simulink model "SSN_39busRT_Ctrl_4WT_19B"  (R2021a)
settings: Solver=ode3  StartTime=0.0  StopTime=10  FixedStep=Ts  MaxStep=1/60  RelTol=1e-2  AbsTol=1e-1
PreLoadFcn:
  | Ts=2.50e-6; ssn_ieee39_params; load('Pwf.mat');
InitFcn:
  | Ts=2.50e-6; ssn_ieee39_params; load('Pwf.mat');
values from neighbouring files (symbols this model uses):
  f = 50    [ssn_ieee39_params_ctrl.m]
  fNom = f    (= 60)    [ssn_ieee39_params_ctrl.m]
  ILR = 5.02    [ssn_ieee39_params_ctrl.m]
  IQMIN = 0.1    [ssn_ieee39_params_ctrl.m]
  ISCLIM = 1    [ssn_ieee39_params_ctrl.m]
  ITFpu = 1.10    (= 1.1)    [ssn_ieee39_params_ctrl.m]
  K = 1    [ssn_ieee39_params_ctrl.m]
  K1 = 1    [ssn_ieee39_params_ctrl.m]
  K2 = 2    [ssn_ieee39_params_ctrl.m]
  KCL = 1.04    [ssn_ieee39_params_ctrl.m]
  KFB = 0    [ssn_ieee39_params_ctrl.m]
  KFF = 1    [ssn_ieee39_params_ctrl.m]
  KFIX = 1    [ssn_ieee39_params_ctrl.m]
  KG = 1    [ssn_ieee39_params_ctrl.m]
  KIA = 59.91    [ssn_ieee39_params_ctrl.m]
  KIOEX = 0.0303    [ssn_ieee39_params_ctrl.m]
  KIUEX = 0.0303    [ssn_ieee39_params_ctrl.m]
  KIUOEX = 1    [ssn_ieee39_params_ctrl.m]
  KIUUEX = 1    [ssn_ieee39_params_ctrl.m]
  KLR = 22.47    [ssn_ieee39_params_ctrl.m]
  KM = 1    [ssn_ieee39_params_ctrl.m]
  KOEL = 0.24    [ssn_ieee39_params_ctrl.m]
  Kp = 1    [ssn_ieee39_params_ctrl.m]
  KPA = 30    [ssn_ieee39_params_ctrl.m]
  KPOEL = 1    [ssn_ieee39_params_ctrl.m]
  KPOEX = 0    [ssn_ieee39_params_ctrl.m]
  KPUEX = 0    [ssn_ieee39_params_ctrl.m]
  KSCALE = 0.319    [ssn_ieee39_params_ctrl.m]
  KUF = 0    [ssn_ieee39_params_ctrl.m]
  KUI = 0.001    [ssn_ieee39_params_ctrl.m]
  KUL = 0.24    [ssn_ieee39_params_ctrl.m]
  s = 10    [ssn_ieee39_params_ctrl.m]
  TA = 0.01    [ssn_ieee39_params_ctrl.m]
  Tadj = 0    [ssn_ieee39_params_ctrl.m]
  taps = [1 1 1.07 1.07 1.009 1.025 1 1.025 1.025 1.025]*1    [ssn_ieee39_params_ctrl.m]
  TF = 0.02    [ssn_ieee39_params_ctrl.m]
  TG = 0.024    [ssn_ieee39_params_ctrl.m]
  TINV = 0    [ssn_ieee39_params_ctrl.m]
  TIT = 0.1    [ssn_ieee39_params_ctrl.m]
  TL_10_11_len = 14    [ssn_ieee39_params_ctrl.m]
  TL_10_13_len = 14    [ssn_ieee39_params_ctrl.m]
  TL_13_14_len = 32    [ssn_ieee39_params_ctrl.m]
  TL_14_15_len = 70    [ssn_ieee39_params_ctrl.m]
  TL_15_16_len = 31.5    [ssn_ieee39_params_ctrl.m]
  TL_16_17_len = 26    [ssn_ieee39_params_ctrl.m]
  TL_16_19_len = 61    [ssn_ieee39_params_ctrl.m]
  TL_16_21_len = 46    [ssn_ieee39_params_ctrl.m]
  TL_16_24_len = 15    [ssn_ieee39_params_ctrl.m]
  TL_17_18_len = 26    [ssn_ieee39_params_ctrl.m]
  TL_17_27_len = 59    [ssn_ieee39_params_ctrl.m]
  TL_1_2_len = 134    [ssn_ieee39_params_ctrl.m]
  TL_1_39_len = 105    [ssn_ieee39_params_ctrl.m]
  TL_21_22_len = 47    [ssn_ieee39_params_ctrl.m]
  TL_22_23_len = 33    [ssn_ieee39_params_ctrl.m]
  TL_24_23_len = 88    [ssn_ieee39_params_ctrl.m]
  TL_25_26_len = 101    [ssn_ieee39_params_ctrl.m]
  TL_26_27_len = 46.5    [ssn_ieee39_params_ctrl.m]
  TL_26_28_len = 151    [ssn_ieee39_params_ctrl.m]
  TL_26_29_len = 200    [ssn_ieee39_params_ctrl.m]
  TL_28_29_len = 48    [ssn_ieee39_params_ctrl.m]
  TL_2_25_len = 28    [ssn_ieee39_params_ctrl.m]
  TL_2_2_len = 49    [ssn_ieee39_params_ctrl.m]
  TL_3_18_len = 42    [ssn_ieee39_params_ctrl.m]
  TL_3_4_len = 53    [ssn_ieee39_params_ctrl.m]
  TL_4_14_len = 33    [ssn_ieee39_params_ctrl.m]
  TL_4_5_len = 32.5    [ssn_ieee39_params_ctrl.m]
  TL_5_6_len = 14    [ssn_ieee39_params_ctrl.m]
  TL_5_8_len = 32    [ssn_ieee39_params_ctrl.m]
  TL_6_11_len = 26.5    [ssn_ieee39_params_ctrl.m]
  TL_6_7_len = 25.5    [ssn_ieee39_params_ctrl.m]
  TL_7_8_len = 15    [ssn_ieee39_params_ctrl.m]
  TL_8_9_len = 93    [ssn_ieee39_params_ctrl.m]
  TL_9_39_len = 136    [ssn_ieee39_params_ctrl.m]
  TOEL = 5.00    (= 5)    [ssn_ieee39_params_ctrl.m]
  TQREF = 0    [ssn_ieee39_params_ctrl.m]
  TQSCL = 0.012    [ssn_ieee39_params_ctrl.m]
  Ts_PMU = 1/1000    (= 0.001)    [ssn_ieee39_params_ctrl.m]
  TU1 = 0    [ssn_ieee39_params_ctrl.m]
  TU2 = 0    [ssn_ieee39_params_ctrl.m]
  TU3 = 0    [ssn_ieee39_params_ctrl.m]
  TU4 = 0    [ssn_ieee39_params_ctrl.m]
  TUL = 0    [ssn_ieee39_params_ctrl.m]
  TUP = 0.050    (= 0.05)    [ssn_ieee39_params_ctrl.m]
  TUQ = .005    (= 0.005)    [ssn_ieee39_params_ctrl.m]
  TUV = 0.2    [ssn_ieee39_params_ctrl.m]
  VAAMAX = VAMAX    (= 7.05)    [ssn_ieee39_params_ctrl.m]
  VAMAX = 7.05    [ssn_ieee39_params_ctrl.m]
  VAMIN = -6.11    [ssn_ieee39_params_ctrl.m]
  VBMAX = 999    [ssn_ieee39_params_ctrl.m]
  VF = 0    [ssn_ieee39_params_ctrl.m]
  VFB = 0    [ssn_ieee39_params_ctrl.m]
  VMMAX = 7.05    [ssn_ieee39_params_ctrl.m]
  VMMIN = -6.11    [ssn_ieee39_params_ctrl.m]
  VOELmax1 = 0.2353    [ssn_ieee39_params_ctrl.m]
  VOELmax2 = 0.0    (= 0)    [ssn_ieee39_params_ctrl.m]
  VOELmin1 = -0.24    [ssn_ieee39_params_ctrl.m]
  VOELmin2 = -1.0    (= -1)    [ssn_ieee39_params_ctrl.m]
  VRMAX = 7.05    [ssn_ieee39_params_ctrl.m]
  VRMIN = -6.11    [ssn_ieee39_params_ctrl.m]
  VSCLmax = 0.20    (= 0.2)    [ssn_ieee39_params_ctrl.m]
  VSCLmin = -0.10    (= -0.1)    [ssn_ieee39_params_ctrl.m]
  VUELmax1 = 1    [ssn_ieee39_params_ctrl.m]
  VUELmax2 = 1    [ssn_ieee39_params_ctrl.m]
  VUELmin1 = -1    [ssn_ieee39_params_ctrl.m]
  VUELmin2 = -1    [ssn_ieee39_params_ctrl.m]
  VUImax = 1    [ssn_ieee39_params_ctrl.m]
  VUImin = -1    [ssn_ieee39_params_ctrl.m]
undefined symbols (not defined in the file or in its folder): another_event_name, D1, Delta, DiscIntNeverNeededParam, find_system, MOV_segment9, my_event_name, powergui, Pw1, Pw2, Pw3, Pw4, vNomHV
libraries: powerlib_extras x162, spsThreePhaseVIMeasurementLib x55, spsCurrentMeasurementLib x52, simulink_extras x44, slpidlib x40, op_dpl_lib x36, spsST2AModel x20, spsThreePhaseParallelRLCLoadLib x20, spsThreePhaseTransformerTwoWindingsLib x17, spsControlledVoltageSourceLib x16, spsVoltageMeasurementLib x12, spsSynchronousMachinepuStandardLib x10
(part 16 of 19)

== system SSN_39busRT_Ctrl_4WT_19B/SM_master/4 WT/SS_windfarm3to4/Wind Farm (DFIG Type)/Wind Turbine Doubly-Fed Induction Generator (Average Model)1/Average_VSC/Converter_model ==
  note: P = Vab*Ia -Vbc*Ic = Vdc*Idc
      | Idc = (Vab*Ia -Vbc*Ic)/Vdc
  Ia_Ic : Inport
  Vdc : Inport  Port=2
  Uref : Inport  Port=3
  Add : Sum  Inputs=+-
  Add1 : Sum  Inputs=+-
  Constant : Constant  Value=1e-6
  Delay1 : UnitDelay  SampleTime=Ts  HasFrameUpgradeWarning=on
  Delay2 : UnitDelay  InitialCondition=1e-6  SampleTime=Ts  HasFrameUpgradeWarning=on
  Demux : Demux  Outputs=3
  Demux1 : Demux  Outputs=2
  Gain : Gain  Gain=0.5
  Mult : Product  Inputs=**
  Mux1 : Mux  Inputs=2
  Predictor : Subsystem
  Product3 : Product  RndMeth=Zero
  Product4 : Product  RndMeth=Zero
  Product5 : Product  Inputs=*/  RndMeth=Zero
  Subtract2 : Sum  Inputs=+-
  Subtract3 : Sum
  Idc : Outport
  Vab_Vbc : Outport  Port=2
  wires:
  Delay1/1 -> Gain/1, Predictor/1(In)
  Gain/1 -> Mult/2
  Mult/1 -> Demux/1
  Demux/3 -> Add1/2
  Demux/2 -> Add/2, Add1/1
  Demux/1 -> Add/1
  Predictor/1(Out) -> Subtract3/1
  Add/1 -> Mux1/1, Product3/1  "Vab"
  Add1/1 -> Mux1/2, Product4/1  "Vbc"
  Demux1/2 -> Product4/2  "ic"
  Product3/1 -> Subtract2/1
  Product4/1 -> Subtract2/2
  Subtract3/1 -> Product5/2
  Constant/1 -> Subtract3/2
  Product5/1 -> Delay2/1
  Subtract2/1 -> Product5/1  "Pac"
  Demux1/1 -> Product3/2  "ia"
  Delay2/1 -> Idc/1  "idc"
  Ia_Ic/1 -> Demux1/1
  Vdc/1 -> Delay1/1
  Uref/1 -> Mult/1
  Mux1/1 -> Vab_Vbc/1

== system SSN_39busRT_Ctrl_4WT_19B/SM_master/4 WT/SS_windfarm3to4/Wind Farm (DFIG Type)/Wind Turbine Doubly-Fed Induction Generator (Average Model)1/Average_VSC1/Converter_model ==
  note: P = Vab*Ia -Vbc*Ic = Vdc*Idc
      | Idc = (Vab*Ia -Vbc*Ic)/Vdc
  Ia_Ic : Inport
  Vdc : Inport  Port=2
  Uref : Inport  Port=3
  Add : Sum  Inputs=+-
  Add1 : Sum  Inputs=+-
  Constant : Constant  Value=1e-6
  Delay1 : UnitDelay  SampleTime=Ts  HasFrameUpgradeWarning=on
  Delay2 : UnitDelay  InitialCondition=1e-6  SampleTime=Ts  HasFrameUpgradeWarning=on
  Demux : Demux  Outputs=3
  Demux1 : Demux  Outputs=2
  Gain : Gain  Gain=0.5
  Mult : Product  Inputs=**
  Mux1 : Mux  Inputs=2
  Predictor : Subsystem
  Product3 : Product  RndMeth=Zero
  Product4 : Product  RndMeth=Zero
  Product5 : Product  Inputs=*/  RndMeth=Zero
  Subtract2 : Sum  Inputs=+-
  Subtract3 : Sum
  Idc : Outport
  Vab_Vbc : Outport  Port=2
  wires:
  Delay1/1 -> Gain/1, Predictor/1(In)
  Gain/1 -> Mult/2
  Mult/1 -> Demux/1
  Demux/3 -> Add1/2
  Demux/2 -> Add/2, Add1/1
  Demux/1 -> Add/1
  Predictor/1(Out) -> Subtract3/1
  Add/1 -> Mux1/1, Product3/1  "Vab"
  Add1/1 -> Mux1/2, Product4/1  "Vbc"
  Demux1/2 -> Product4/2  "ic"
  Product3/1 -> Subtract2/1
  Product4/1 -> Subtract2/2
  Subtract3/1 -> Product5/2
  Constant/1 -> Subtract3/2
  Product5/1 -> Delay2/1
  Subtract2/1 -> Product5/1  "Pac"
  Demux1/1 -> Product3/2  "ia"
  Delay2/1 -> Idc/1  "idc"
  Ia_Ic/1 -> Demux1/1
  Vdc/1 -> Delay1/1
  Uref/1 -> Mult/1
  Mux1/1 -> Vab_Vbc/1

== system SSN_39busRT_Ctrl_4WT_19B/SM_master/4 WT/SS_windfarm3to4/Wind Farm (DFIG Type)/Wind Turbine Doubly-Fed Induction Generator (Average Model)1/Control System_average/Control ==
  Vabc_B1 : Inport
  Iabc_grid_conv : Inport  Port=2
  Vdc : Inport  Port=3
  Iabc_stator : Inport  Port=4
  Iabc_rotor : Inport  Port=5
  Q_ref : Inport  Port=6
  Iq_grid_conv_ref : Inport  Port=7
  Q_B1 : Inport  Port=8
  wr : Inport  Port=9
  angle_rotor : Inport  Port=10
  0-pitch_max : Saturate  UpperLimit=pitch_max  LowerLimit=0
  Constant2 : Constant  Value=speed_D
  Discrete 3-phase PLL : powerlib_extras/Discrete  Control Blocks/Discrete 3-phase PLL  Fmin=Fnom-10  Par_Init=[-45 Fnom]  ParK=[60 1400]  Ts=Ts  AGC=off
      settings: SourceProductBaseCode=PS
  Grid-side converter Control system : Subsystem
  Mux : Mux  Inputs=2
  "Rate Limiter   " : RateLimiter  RisingSlewLimit=pitch_rate  FallingSlewLimit=-pitch_rate
  Rotor-side converter Control system : Subsystem
  Sum : Sum  Inputs=|+-  SaturateOnIntegerOverflow=on
  Terminator : Terminator
  pitch_gain : Gain  Gain=pitch_gain  SaturateOnIntegerOverflow=on  OutDataTypeStr=Inherit: Same as input  ParamDataTypeStr=Inherit: Same as input
  Uctrl_grid_conv : Outport
  Uctrl_rotor_conv : Outport  Port=2
  Theta_Freq : Outport  Port=3
  Pitch_angle : Outport  Port=4
  wires:
  Vdc/1 -> Grid-side converter Control system/4(Vdc), Rotor-side converter Control system/2(Vdc)
  Vabc_B1/1 -> Grid-side converter Control system/1(Vabc_B1), Discrete 3-phase PLL/1
  Iq_grid_conv_ref/1 -> Grid-side converter Control system/5(Iq_ref)
  Iabc_grid_conv/1 -> Grid-side converter Control system/2(Iabc_grid_conv), Rotor-side converter Control system/6(Iabc_grid_conv)
  Iabc_stator/1 -> Rotor-side converter Control system/4(Iabc_stator)
  Iabc_rotor/1 -> Rotor-side converter Control system/5(Iabc_rotor)
  Q_ref/1 -> Rotor-side converter Control system/7(Q_ref)
  Discrete 3-phase PLL/2 -> Grid-side converter Control system/3(Theta), Mux/1, Rotor-side converter Control system/3(Theta)
  Mux/1 -> Theta_Freq/1
  Discrete 3-phase PLL/3 -> Terminator/1
  Discrete 3-phase PLL/1 -> Grid-side converter Control system/6(Freq), Mux/2, Rotor-side converter Control system/10(Freq)
  "Rate Limiter   "/1 -> Pitch_angle/1
  pitch_gain/1 -> 0-pitch_max/1
  Sum/1 -> pitch_gain/1
  Constant2/1 -> Sum/2
  0-pitch_max/1 -> "Rate Limiter   "/1
  wr/1 -> Sum/1, Rotor-side converter Control system/1(wr)
  Q_B1/1 -> Rotor-side converter Control system/8(Q_B1)
  angle_rotor/1 -> Rotor-side converter Control system/9(angle_rotor)
  Grid-side converter Control system/2(Vdqs) -> [Vdqs]
  [Vdqs] -> Rotor-side converter Control system/11(Vdqs)
  Grid-side converter Control system/1(Uctrl_grid_conv) -> Uctrl_grid_conv/1
  Rotor-side converter Control system/1(Uctrl_rotor_conv) -> Uctrl_rotor_conv/1

== system SSN_39busRT_Ctrl_4WT_19B/SM_master/4 WT/SS_windfarm3to4/Wind Farm (DFIG Type)/Wind Turbine Doubly-Fed Induction Generator (Average Model)1/Control System_average/Filter 1000 Hz ==
  Vabc_B1 : Inport
  Iabc_grid_conv : Inport  Port=2
  Vdc : Inport  Port=3
  Iabc_stator : Inport  Port=4
  Iabc_rotor : Inport  Port=5
  Q_ref : Inport  Port=6
  Iq_grid_conv_ref : Inport  Port=7
  Q_B1 : Inport  Port=8
  wr : Inport  Port=9
  angle_rotor : Inport  Port=10
  Demux{,1..3} (4 alike) : Demux  Outputs=3
      settings: DisplayOption=none
  Discrete 2nd-Order Filter{1..14,16..18,20} (18 alike) : powerlib_extras/Discrete  Control Blocks/Discrete  2nd-Order Filter  FilterType=Lowpass  Fo=Freq  Zeta=Zeta  Ts=Ts  Initialize=off  Vac_Init=[0.8 -25 60]  Vdc_Init=-0.4  PlotResponse=off  param1=[1 500 1]
      settings: SourceProductBaseCode=PS
  Mux{,1..3} (4 alike) : Mux  Inputs=3
  "Vabc_B1 " : Outport
  "Iabc_grid_conv " : Outport  Port=2
  "Vdc " : Outport  Port=3
  "Iabc_stator " : Outport  Port=4
  "Iabc_rotor " : Outport  Port=5
  "Q_ref " : Outport  Port=6
  "Iq_grid_conv_ref " : Outport  Port=7
  "Q_B1 " : Outport  Port=8
  "wr " : Outport  Port=9
  "angle_rotor " : Outport  Port=10
  wires:
  Demux/1 -> Discrete 2nd-Order Filter1/1
  Demux/2 -> Discrete 2nd-Order Filter2/1
  Demux/3 -> Discrete 2nd-Order Filter3/1
  Discrete 2nd-Order Filter1/1 -> Mux/1
  Discrete 2nd-Order Filter2/1 -> Mux/2
  Discrete 2nd-Order Filter3/1 -> Mux/3
  Vabc_B1/1 -> Demux/1
  Mux/1 -> "Vabc_B1 "/1
  Demux1/1 -> Discrete 2nd-Order Filter4/1
  Demux1/2 -> Discrete 2nd-Order Filter5/1
  Demux1/3 -> Discrete 2nd-Order Filter6/1
  Discrete 2nd-Order Filter4/1 -> Mux1/1
  Discrete 2nd-Order Filter5/1 -> Mux1/2
  Discrete 2nd-Order Filter6/1 -> Mux1/3
  Iabc_grid_conv/1 -> Demux1/1
  Mux1/1 -> "Iabc_grid_conv "/1
  Vdc/1 -> Discrete 2nd-Order Filter7/1
  Discrete 2nd-Order Filter7/1 -> "Vdc "/1
  Demux2/1 -> Discrete 2nd-Order Filter8/1
  Demux2/2 -> Discrete 2nd-Order Filter9/1
  Demux2/3 -> Discrete 2nd-Order Filter10/1
  Discrete 2nd-Order Filter8/1 -> Mux2/1
  Discrete 2nd-Order Filter9/1 -> Mux2/2
  Discrete 2nd-Order Filter10/1 -> Mux2/3
  Iabc_stator/1 -> Demux2/1
  Mux2/1 -> "Iabc_stator "/1
  Q_ref/1 -> Discrete 2nd-Order Filter11/1
  Q_B1/1 -> Discrete 2nd-Order Filter12/1
  Discrete 2nd-Order Filter12/1 -> "Q_B1 "/1
  wr/1 -> Discrete 2nd-Order Filter13/1
  Discrete 2nd-Order Filter13/1 -> "wr "/1
  angle_rotor/1 -> Discrete 2nd-Order Filter14/1
  Discrete 2nd-Order Filter14/1 -> "angle_rotor "/1
  Discrete 2nd-Order Filter11/1 -> "Q_ref "/1
  Demux3/1 -> Discrete 2nd-Order Filter17/1
  Demux3/2 -> Discrete 2nd-Order Filter18/1
  Demux3/3 -> Discrete 2nd-Order Filter16/1
  Discrete 2nd-Order Filter17/1 -> Mux3/1
  Discrete 2nd-Order Filter18/1 -> Mux3/2
  Discrete 2nd-Order Filter16/1 -> Mux3/3
  Iabc_rotor/1 -> Demux3/1
  Mux3/1 -> "Iabc_rotor "/1
  Iq_grid_conv_ref/1 -> Discrete 2nd-Order Filter20/1
  Discrete 2nd-Order Filter20/1 -> "Iq_grid_conv_ref "/1

== system SSN_39busRT_Ctrl_4WT_19B/SM_master/4 WT/SS_windfarm3to4/Wind Farm (DFIG Type)2/Wind Turbine Doubly-Fed Induction Generator (Average Model)1/Average_VSC/Converter_model ==
  note: P = Vab*Ia -Vbc*Ic = Vdc*Idc
      | Idc = (Vab*Ia -Vbc*Ic)/Vdc
  Ia_Ic : Inport
  Vdc : Inport  Port=2
  Uref : Inport  Port=3
  Add : Sum  Inputs=+-
  Add1 : Sum  Inputs=+-
  Constant : Constant  Value=1e-6
  Delay1 : UnitDelay  SampleTime=Ts  HasFrameUpgradeWarning=on
  Delay2 : UnitDelay  InitialCondition=1e-6  SampleTime=Ts  HasFrameUpgradeWarning=on
  Demux : Demux  Outputs=3
  Demux1 : Demux  Outputs=2
  Gain : Gain  Gain=0.5
  Mult : Product  Inputs=**
  Mux1 : Mux  Inputs=2
  Predictor : Subsystem
  Product3 : Product  RndMeth=Zero
  Product4 : Product  RndMeth=Zero
  Product5 : Product  Inputs=*/  RndMeth=Zero
  Subtract2 : Sum  Inputs=+-
  Subtract3 : Sum
  Idc : Outport
  Vab_Vbc : Outport  Port=2
  wires:
  Mux1/1 -> Vab_Vbc/1
  Uref/1 -> Mult/1
  Vdc/1 -> Delay1/1
  Ia_Ic/1 -> Demux1/1
  Delay2/1 -> Idc/1  "idc"
  Demux1/1 -> Product3/2  "ia"
  Subtract2/1 -> Product5/1  "Pac"
  Product5/1 -> Delay2/1
  Constant/1 -> Subtract3/2
  Subtract3/1 -> Product5/2
  Product4/1 -> Subtract2/2
  Product3/1 -> Subtract2/1
  Demux1/2 -> Product4/2  "ic"
  Add1/1 -> Product4/1, Mux1/2  "Vbc"
  Add/1 -> Product3/1, Mux1/1  "Vab"
  Predictor/1(Out) -> Subtract3/1
  Demux/1 -> Add/1
  Demux/2 -> Add1/1, Add/2
  Demux/3 -> Add1/2
  Mult/1 -> Demux/1
  Gain/1 -> Mult/2
  Delay1/1 -> Predictor/1(In), Gain/1

== system SSN_39busRT_Ctrl_4WT_19B/SM_master/4 WT/SS_windfarm3to4/Wind Farm (DFIG Type)2/Wind Turbine Doubly-Fed Induction Generator (Average Model)1/Average_VSC1/Converter_model ==
  note: P = Vab*Ia -Vbc*Ic = Vdc*Idc
      | Idc = (Vab*Ia -Vbc*Ic)/Vdc
  Ia_Ic : Inport
  Vdc : Inport  Port=2
  Uref : Inport  Port=3
  Add : Sum  Inputs=+-
  Add1 : Sum  Inputs=+-
  Constant : Constant  Value=1e-6
  Delay1 : UnitDelay  SampleTime=Ts  HasFrameUpgradeWarning=on
  Delay2 : UnitDelay  InitialCondition=1e-6  SampleTime=Ts  HasFrameUpgradeWarning=on
  Demux : Demux  Outputs=3
  Demux1 : Demux  Outputs=2
  Gain : Gain  Gain=0.5
  Mult : Product  Inputs=**
  Mux1 : Mux  Inputs=2
  Predictor : Subsystem
  Product3 : Product  RndMeth=Zero
  Product4 : Product  RndMeth=Zero
  Product5 : Product  Inputs=*/  RndMeth=Zero
  Subtract2 : Sum  Inputs=+-
  Subtract3 : Sum
  Idc : Outport
  Vab_Vbc : Outport  Port=2
  wires:
  Mux1/1 -> Vab_Vbc/1
  Uref/1 -> Mult/1
  Vdc/1 -> Delay1/1
  Ia_Ic/1 -> Demux1/1
  Delay2/1 -> Idc/1  "idc"
  Demux1/1 -> Product3/2  "ia"
  Subtract2/1 -> Product5/1  "Pac"
  Product5/1 -> Delay2/1
  Constant/1 -> Subtract3/2
  Subtract3/1 -> Product5/2
  Product4/1 -> Subtract2/2
  Product3/1 -> Subtract2/1
  Demux1/2 -> Product4/2  "ic"
  Add1/1 -> Product4/1, Mux1/2  "Vbc"
  Add/1 -> Product3/1, Mux1/1  "Vab"
  Predictor/1(Out) -> Subtract3/1
  Demux/1 -> Add/1
  Demux/2 -> Add1/1, Add/2
  Demux/3 -> Add1/2
  Mult/1 -> Demux/1
  Gain/1 -> Mult/2
  Delay1/1 -> Predictor/1(In), Gain/1

== system SSN_39busRT_Ctrl_4WT_19B/SM_master/4 WT/SS_windfarm3to4/Wind Farm (DFIG Type)2/Wind Turbine Doubly-Fed Induction Generator (Average Model)1/Control System_average/Control ==
  Vabc_B1 : Inport
  Iabc_grid_conv : Inport  Port=2
  Vdc : Inport  Port=3
  Iabc_stator : Inport  Port=4
  Iabc_rotor : Inport  Port=5
  Q_ref : Inport  Port=6
  Iq_grid_conv_ref : Inport  Port=7
  Q_B1 : Inport  Port=8
  wr : Inport  Port=9
  angle_rotor : Inport  Port=10
  0-pitch_max : Saturate  UpperLimit=pitch_max  LowerLimit=0
  Constant2 : Constant  Value=speed_D
  Discrete 3-phase PLL : powerlib_extras/Discrete  Control Blocks/Discrete 3-phase PLL  Fmin=Fnom-10  Par_Init=[-45 Fnom]  ParK=[60 1400]  Ts=Ts  AGC=off
      settings: SourceProductBaseCode=PS
  Grid-side converter Control system : Subsystem
  Mux : Mux  Inputs=2
  "Rate Limiter   " : RateLimiter  RisingSlewLimit=pitch_rate  FallingSlewLimit=-pitch_rate
  Rotor-side converter Control system : Subsystem
  Sum : Sum  Inputs=|+-  SaturateOnIntegerOverflow=on
  Terminator : Terminator
  pitch_gain : Gain  Gain=pitch_gain  SaturateOnIntegerOverflow=on  OutDataTypeStr=Inherit: Same as input  ParamDataTypeStr=Inherit: Same as input
  Uctrl_grid_conv : Outport
  Uctrl_rotor_conv : Outport  Port=2
  Theta_Freq : Outport  Port=3
  Pitch_angle : Outport  Port=4
  wires:
  Rotor-side converter Control system/1(Uctrl_rotor_conv) -> Uctrl_rotor_conv/1
  Grid-side converter Control system/1(Uctrl_grid_conv) -> Uctrl_grid_conv/1
  [Vdqs] -> Rotor-side converter Control system/11(Vdqs)
  Grid-side converter Control system/2(Vdqs) -> [Vdqs]
  angle_rotor/1 -> Rotor-side converter Control system/9(angle_rotor)
  Q_B1/1 -> Rotor-side converter Control system/8(Q_B1)
  wr/1 -> Rotor-side converter Control system/1(wr), Sum/1
  0-pitch_max/1 -> "Rate Limiter   "/1
  Constant2/1 -> Sum/2
  Sum/1 -> pitch_gain/1
  pitch_gain/1 -> 0-pitch_max/1
  "Rate Limiter   "/1 -> Pitch_angle/1
  Discrete 3-phase PLL/1 -> Rotor-side converter Control system/10(Freq), Mux/2, Grid-side converter Control system/6(Freq)
  Discrete 3-phase PLL/3 -> Terminator/1
  Mux/1 -> Theta_Freq/1
  Discrete 3-phase PLL/2 -> Rotor-side converter Control system/3(Theta), Mux/1, Grid-side converter Control system/3(Theta)
  Q_ref/1 -> Rotor-side converter Control system/7(Q_ref)
  Iabc_rotor/1 -> Rotor-side converter Control system/5(Iabc_rotor)
  Iabc_stator/1 -> Rotor-side converter Control system/4(Iabc_stator)
  Iabc_grid_conv/1 -> Rotor-side converter Control system/6(Iabc_grid_conv), Grid-side converter Control system/2(Iabc_grid_conv)
  Iq_grid_conv_ref/1 -> Grid-side converter Control system/5(Iq_ref)
  Vabc_B1/1 -> Discrete 3-phase PLL/1, Grid-side converter Control system/1(Vabc_B1)
  Vdc/1 -> Rotor-side converter Control system/2(Vdc), Grid-side converter Control system/4(Vdc)

== system SSN_39busRT_Ctrl_4WT_19B/SM_master/4 WT/SS_windfarm3to4/Wind Farm (DFIG Type)2/Wind Turbine Doubly-Fed Induction Generator (Average Model)1/Control System_average/Filter 1000 Hz ==
  Vabc_B1 : Inport
  Iabc_grid_conv : Inport  Port=2
  Vdc : Inport  Port=3
  Iabc_stator : Inport  Port=4
  Iabc_rotor : Inport  Port=5
  Q_ref : Inport  Port=6
  Iq_grid_conv_ref : Inport  Port=7
  Q_B1 : Inport  Port=8
  wr : Inport  Port=9
  angle_rotor : Inport  Port=10
  Demux{,1..3} (4 alike) : Demux  Outputs=3
      settings: DisplayOption=none
  Discrete 2nd-Order Filter{1..14,16..18,20} (18 alike) : powerlib_extras/Discrete  Control Blocks/Discrete  2nd-Order Filter  FilterType=Lowpass  Fo=Freq  Zeta=Zeta  Ts=Ts  Initialize=off  Vac_Init=[0.8 -25 60]  Vdc_Init=-0.4  PlotResponse=off  param1=[1 500 1]
      settings: SourceProductBaseCode=PS
  Mux{,1..3} (4 alike) : Mux  Inputs=3
  "Vabc_B1 " : Outport
  "Iabc_grid_conv " : Outport  Port=2
  "Vdc " : Outport  Port=3
  "Iabc_stator " : Outport  Port=4
  "Iabc_rotor " : Outport  Port=5
  "Q_ref " : Outport  Port=6
  "Iq_grid_conv_ref " : Outport  Port=7
  "Q_B1 " : Outport  Port=8
  "wr " : Outport  Port=9
  "angle_rotor " : Outport  Port=10
  wires:
  Discrete 2nd-Order Filter20/1 -> "Iq_grid_conv_ref "/1
  Iq_grid_conv_ref/1 -> Discrete 2nd-Order Filter20/1
  Mux3/1 -> "Iabc_rotor "/1
  Iabc_rotor/1 -> Demux3/1
  Discrete 2nd-Order Filter16/1 -> Mux3/3
  Discrete 2nd-Order Filter18/1 -> Mux3/2
  Discrete 2nd-Order Filter17/1 -> Mux3/1
  Demux3/3 -> Discrete 2nd-Order Filter16/1
  Demux3/2 -> Discrete 2nd-Order Filter18/1
  Demux3/1 -> Discrete 2nd-Order Filter17/1
  Discrete 2nd-Order Filter11/1 -> "Q_ref "/1
  Discrete 2nd-Order Filter14/1 -> "angle_rotor "/1
  angle_rotor/1 -> Discrete 2nd-Order Filter14/1
  Discrete 2nd-Order Filter13/1 -> "wr "/1
  wr/1 -> Discrete 2nd-Order Filter13/1
  Discrete 2nd-Order Filter12/1 -> "Q_B1 "/1
  Q_B1/1 -> Discrete 2nd-Order Filter12/1
  Q_ref/1 -> Discrete 2nd-Order Filter11/1
  Mux2/1 -> "Iabc_stator "/1
  Iabc_stator/1 -> Demux2/1
  Discrete 2nd-Order Filter10/1 -> Mux2/3
  Discrete 2nd-Order Filter9/1 -> Mux2/2
  Discrete 2nd-Order Filter8/1 -> Mux2/1
  Demux2/3 -> Discrete 2nd-Order Filter10/1
  Demux2/2 -> Discrete 2nd-Order Filter9/1
  Demux2/1 -> Discrete 2nd-Order Filter8/1
  Discrete 2nd-Order Filter7/1 -> "Vdc "/1
  Vdc/1 -> Discrete 2nd-Order Filter7/1
  Mux1/1 -> "Iabc_grid_conv "/1
  Iabc_grid_conv/1 -> Demux1/1
  Discrete 2nd-Order Filter6/1 -> Mux1/3
  Discrete 2nd-Order Filter5/1 -> Mux1/2
  Discrete 2nd-Order Filter4/1 -> Mux1/1
  Demux1/3 -> Discrete 2nd-Order Filter6/1
  Demux1/2 -> Discrete 2nd-Order Filter5/1
  Demux1/1 -> Discrete 2nd-Order Filter4/1
  Mux/1 -> "Vabc_B1 "/1
  Vabc_B1/1 -> Demux/1
  Discrete 2nd-Order Filter3/1 -> Mux/3
  Discrete 2nd-Order Filter2/1 -> Mux/2
  Discrete 2nd-Order Filter1/1 -> Mux/1
  Demux/3 -> Discrete 2nd-Order Filter3/1
  Demux/2 -> Discrete 2nd-Order Filter2/1
  Demux/1 -> Discrete 2nd-Order Filter1/1

== system SSN_39busRT_Ctrl_4WT_19B/SM_master/4 WT/SS_windfarm1to2/Wind Farm (DFIG Type)/Wind Turbine Doubly-Fed Induction Generator (Average Model)1/Average_VSC/Converter_model/Predictor ==
  In : Inport
  Add2 : Sum  Inputs=+-
  Gain1 : Gain  Gain=2
  Unit Delay : UnitDelay  SampleTime=Ts  HasFrameUpgradeWarning=on
  Out : Outport
  wires:
  In/1 -> Unit Delay/1, Gain1/1
  Gain1/1 -> Add2/1
  Unit Delay/1 -> Add2/2
  Add2/1 -> Out/1

== system SSN_39busRT_Ctrl_4WT_19B/SM_master/4 WT/SS_windfarm1to2/Wind Farm (DFIG Type)/Wind Turbine Doubly-Fed Induction Generator (Average Model)1/Average_VSC1/Converter_model/Predictor ==
  In : Inport
  Add2 : Sum  Inputs=+-
  Gain1 : Gain  Gain=2
  Unit Delay : UnitDelay  SampleTime=Ts  HasFrameUpgradeWarning=on
  Out : Outport
  wires:
  In/1 -> Unit Delay/1, Gain1/1
  Gain1/1 -> Add2/1
  Unit Delay/1 -> Add2/2
  Add2/1 -> Out/1

== system SSN_39busRT_Ctrl_4WT_19B/SM_master/4 WT/SS_windfarm1to2/Wind Farm (DFIG Type)/Wind Turbine Doubly-Fed Induction Generator (Average Model)1/Control System_average/Control/Grid-side converter Control system ==
  note: Grid-side converter control system
  Vabc_B1 : Inport
  Iabc_grid_conv : Inport  Port=2
  Theta : Inport  Port=3
  Vdc : Inport  Port=4
  Iq_ref : Inport  Port=5
  Freq : Inport  Port=6
  Current regulator : Subsystem
  DC bus voltage Regulator : Subsystem
  Idq references : Subsystem
  Mux : Mux  Inputs=2
  Rate Limiter : RateLimiter  RisingSlewLimit=current_slew_rate  FallingSlewLimit=-current_slew_rate
  Subsystem1 : Subsystem
  Transformation abc --> dq : Subsystem
  Vdc_ref (V) : Constant  Value=Vdc_nom
  Uctrl_grid_conv : Outport
  Vdqs : Outport  Port=2
  wires:
  Transformation abc --> dq/1(Vdq) -> Current regulator/1(Vdqs), Vdqs/1
  Theta/1 -> Transformation abc --> dq/1(Theta), Subsystem1/1(Theta)
  Vdc/1 -> Subsystem1/3(Vdc), DC bus voltage Regulator/2(Vdc)
  DC bus voltage Regulator/1(Id_ref) -> Mux/1
  Transformation abc --> dq/2(Idq) -> Current regulator/2(Idq)
  Mux/1 -> Idq references/1(Id*Iq*)
  Rate Limiter/1 -> Mux/2
  Iq_ref/1 -> Rate Limiter/1
  Vabc_B1/1 -> Transformation abc --> dq/2(Vabc)
  Iabc_grid_conv/1 -> Transformation abc --> dq/3(Iabc)
  Subsystem1/1(Uctrl_grid_conv) -> Uctrl_grid_conv/1
  Vdc_ref (V)/1 -> DC bus voltage Regulator/1(Vdc_ref)
  Current regulator/1(Vdq*) -> Subsystem1/2(Vdq*)
  Idq references/1(Idq_ref) -> Current regulator/4(Idq_ref)
  Freq/1 -> Current regulator/3(Freq)

== system SSN_39busRT_Ctrl_4WT_19B/SM_master/4 WT/SS_windfarm1to2/Wind Farm (DFIG Type)/Wind Turbine Doubly-Fed Induction Generator (Average Model)1/Control System_average/Control/Rotor-side converter Control system ==
  note: Rotor-side converter control system
  wr : Inport
  Vdc : Inport  Port=2
  Theta : Inport  Port=3
  Iabc_stator : Inport  Port=4
  Iabc_rotor : Inport  Port=5
  Iabc_grid_conv : Inport  Port=6
  Q_ref : Inport  Port=7
  Q_B1 : Inport  Port=8
  angle_rotor : Inport  Port=9
  Freq : Inport  Port=10
  Vdqs : Inport  Port=11
  Current Regulator : Subsystem
  Mux3 : Mux  Inputs=2
  Priority Iqr : Subsystem
  Q Regulator : Subsystem
  Torque control : Subsystem
  "Transformation abc --> dq " : Subsystem
  dq --> abc : Subsystem
  Uctrl_rotor_conv : Outport
  wires:
  Current Regulator/1(Vdq*) -> dq --> abc/1(Vdq*)
  Vdc/1 -> dq --> abc/2(Vdc)
  Theta/1 -> "Transformation abc --> dq "/1(Theta)
  dq --> abc/1(Uctrl_rotor_conv) -> Uctrl_rotor_conv/1
  Iabc_rotor/1 -> "Transformation abc --> dq "/2(Iabc_r)
  Iabc_stator/1 -> "Transformation abc --> dq "/3(Iabc_s)
  Iabc_grid_conv/1 -> "Transformation abc --> dq "/4(Iabc_grid_conv)
  "Transformation abc --> dq "/1(Idq_r) -> Current Regulator/2(Idq_r), Torque control/2(Idqr)
  "Transformation abc --> dq "/2(Idq_s) -> Torque control/3(Idqs), Current Regulator/3(Idq_s)
  angle_rotor/1 -> "Transformation abc --> dq "/5(angle_rotor)
  Mux3/1 -> Priority Iqr/1(Idqr*)
  "Transformation abc --> dq "/4(r_angle_transformation) -> dq --> abc/3(Angle)
  Freq/1 -> Torque control/5(Freq), Current Regulator/5(Freq)
  wr/1 -> Torque control/1(wr), Current Regulator/4(wr)
  "Transformation abc --> dq "/3(Idq_gc) -> Torque control/4(Idq_grid_conv)
  Vdqs/1 -> Torque control/6(Vdqs)
  Q_ref/1 -> Q Regulator/1(Q_ref)
  Q_B1/1 -> Q Regulator/2(Q_B1)
  Torque control/1(Idr*) -> Mux3/1
  Q Regulator/1(Iqr*) -> Mux3/2
  Priority Iqr/1(Idqr_ref) -> Current Regulator/1(Idqr_ref)

== system SSN_39busRT_Ctrl_4WT_19B/SM_master/4 WT/SS_windfarm1to2/Wind Farm (DFIG Type)1/Wind Turbine Doubly-Fed Induction Generator (Average Model)1/Average_VSC/Converter_model/Predictor ==
  In : Inport
  Add2 : Sum  Inputs=+-
  Gain1 : Gain  Gain=2
  Unit Delay : UnitDelay  SampleTime=Ts  HasFrameUpgradeWarning=on
  Out : Outport
  wires:
  Add2/1 -> Out/1
  Unit Delay/1 -> Add2/2
  Gain1/1 -> Add2/1
  In/1 -> Gain1/1, Unit Delay/1

== system SSN_39busRT_Ctrl_4WT_19B/SM_master/4 WT/SS_windfarm1to2/Wind Farm (DFIG Type)1/Wind Turbine Doubly-Fed Induction Generator (Average Model)1/Average_VSC1/Converter_model/Predictor ==
  In : Inport
  Add2 : Sum  Inputs=+-
  Gain1 : Gain  Gain=2
  Unit Delay : UnitDelay  SampleTime=Ts  HasFrameUpgradeWarning=on
  Out : Outport
  wires:
  Add2/1 -> Out/1
  Unit Delay/1 -> Add2/2
  Gain1/1 -> Add2/1
  In/1 -> Gain1/1, Unit Delay/1

== system SSN_39busRT_Ctrl_4WT_19B/SM_master/4 WT/SS_windfarm1to2/Wind Farm (DFIG Type)1/Wind Turbine Doubly-Fed Induction Generator (Average Model)1/Control System_average/Control/Grid-side converter Control system ==
  note: Grid-side converter control system
  Vabc_B1 : Inport
  Iabc_grid_conv : Inport  Port=2
  Theta : Inport  Port=3
  Vdc : Inport  Port=4
  Iq_ref : Inport  Port=5
  Freq : Inport  Port=6
  Current regulator : Subsystem
  DC bus voltage Regulator : Subsystem
  Idq references : Subsystem
  Mux : Mux  Inputs=2
  Rate Limiter : RateLimiter  RisingSlewLimit=current_slew_rate  FallingSlewLimit=-current_slew_rate
  Subsystem1 : Subsystem
  Transformation abc --> dq : Subsystem
  Vdc_ref (V) : Constant  Value=Vdc_nom
  Uctrl_grid_conv : Outport
  Vdqs : Outport  Port=2
  wires:
  Freq/1 -> Current regulator/3(Freq)
  Idq references/1(Idq_ref) -> Current regulator/4(Idq_ref)
  Current regulator/1(Vdq*) -> Subsystem1/2(Vdq*)
  Vdc_ref (V)/1 -> DC bus voltage Regulator/1(Vdc_ref)
  Subsystem1/1(Uctrl_grid_conv) -> Uctrl_grid_conv/1
  Iabc_grid_conv/1 -> Transformation abc --> dq/3(Iabc)
  Vabc_B1/1 -> Transformation abc --> dq/2(Vabc)
  Iq_ref/1 -> Rate Limiter/1
  Rate Limiter/1 -> Mux/2
  Mux/1 -> Idq references/1(Id*Iq*)
  Transformation abc --> dq/2(Idq) -> Current regulator/2(Idq)
  DC bus voltage Regulator/1(Id_ref) -> Mux/1
  Vdc/1 -> DC bus voltage Regulator/2(Vdc), Subsystem1/3(Vdc)
  Theta/1 -> Subsystem1/1(Theta), Transformation abc --> dq/1(Theta)
  Transformation abc --> dq/1(Vdq) -> Vdqs/1, Current regulator/1(Vdqs)

== system SSN_39busRT_Ctrl_4WT_19B/SM_master/4 WT/SS_windfarm1to2/Wind Farm (DFIG Type)1/Wind Turbine Doubly-Fed Induction Generator (Average Model)1/Control System_average/Control/Rotor-side converter Control system ==
  note: Rotor-side converter control system
  wr : Inport
  Vdc : Inport  Port=2
  Theta : Inport  Port=3
  Iabc_stator : Inport  Port=4
  Iabc_rotor : Inport  Port=5
  Iabc_grid_conv : Inport  Port=6
  Q_ref : Inport  Port=7
  Q_B1 : Inport  Port=8
  angle_rotor : Inport  Port=9
  Freq : Inport  Port=10
  Vdqs : Inport  Port=11
  Current Regulator : Subsystem
  Mux3 : Mux  Inputs=2
  Priority Iqr : Subsystem
  Q Regulator : Subsystem
  Torque control : Subsystem
  "Transformation abc --> dq " : Subsystem
  dq --> abc : Subsystem
  Uctrl_rotor_conv : Outport
  wires:
  Priority Iqr/1(Idqr_ref) -> Current Regulator/1(Idqr_ref)
  Q Regulator/1(Iqr*) -> Mux3/2
  Torque control/1(Idr*) -> Mux3/1
  Q_B1/1 -> Q Regulator/2(Q_B1)
  Q_ref/1 -> Q Regulator/1(Q_ref)
  Vdqs/1 -> Torque control/6(Vdqs)
  "Transformation abc --> dq "/3(Idq_gc) -> Torque control/4(Idq_grid_conv)
  wr/1 -> Current Regulator/4(wr), Torque control/1(wr)
  Freq/1 -> Current Regulator/5(Freq), Torque control/5(Freq)
  "Transformation abc --> dq "/4(r_angle_transformation) -> dq --> abc/3(Angle)
  Mux3/1 -> Priority Iqr/1(Idqr*)
  angle_rotor/1 -> "Transformation abc --> dq "/5(angle_rotor)
  "Transformation abc --> dq "/2(Idq_s) -> Current Regulator/3(Idq_s), Torque control/3(Idqs)
  "Transformation abc --> dq "/1(Idq_r) -> Torque control/2(Idqr), Current Regulator/2(Idq_r)
  Iabc_grid_conv/1 -> "Transformation abc --> dq "/4(Iabc_grid_conv)
  Iabc_stator/1 -> "Transformation abc --> dq "/3(Iabc_s)
  Iabc_rotor/1 -> "Transformation abc --> dq "/2(Iabc_r)
  dq --> abc/1(Uctrl_rotor_conv) -> Uctrl_rotor_conv/1
  Theta/1 -> "Transformation abc --> dq "/1(Theta)
  Vdc/1 -> dq --> abc/2(Vdc)
  Current Regulator/1(Vdq*) -> dq --> abc/1(Vdq*)

== system SSN_39busRT_Ctrl_4WT_19B/SM_master/4 WT/SS_windfarm3to4/Wind Farm (DFIG Type)/Wind Turbine Doubly-Fed Induction Generator (Average Model)1/Average_VSC/Converter_model/Predictor ==
  In : Inport
  Add2 : Sum  Inputs=+-
  Gain1 : Gain  Gain=2
  Unit Delay : UnitDelay  SampleTime=Ts  HasFrameUpgradeWarning=on
  Out : Outport
  wires:
  In/1 -> Unit Delay/1, Gain1/1
  Gain1/1 -> Add2/1
  Unit Delay/1 -> Add2/2
  Add2/1 -> Out/1

== system SSN_39busRT_Ctrl_4WT_19B/SM_master/4 WT/SS_windfarm3to4/Wind Farm (DFIG Type)/Wind Turbine Doubly-Fed Induction Generator (Average Model)1/Average_VSC1/Converter_model/Predictor ==
  In : Inport
  Add2 : Sum  Inputs=+-
  Gain1 : Gain  Gain=2
  Unit Delay : UnitDelay  SampleTime=Ts  HasFrameUpgradeWarning=on
  Out : Outport
  wires:
  In/1 -> Unit Delay/1, Gain1/1
  Gain1/1 -> Add2/1
  Unit Delay/1 -> Add2/2
  Add2/1 -> Out/1

== system SSN_39busRT_Ctrl_4WT_19B/SM_master/4 WT/SS_windfarm3to4/Wind Farm (DFIG Type)/Wind Turbine Doubly-Fed Induction Generator (Average Model)1/Control System_average/Control/Grid-side converter Control system ==
  note: Grid-side converter control system
  Vabc_B1 : Inport
  Iabc_grid_conv : Inport  Port=2
  Theta : Inport  Port=3
  Vdc : Inport  Port=4
  Iq_ref : Inport  Port=5
  Freq : Inport  Port=6
  Current regulator : Subsystem
  DC bus voltage Regulator : Subsystem
  Idq references : Subsystem
  Mux : Mux  Inputs=2
  Rate Limiter : RateLimiter  RisingSlewLimit=current_slew_rate  FallingSlewLimit=-current_slew_rate
  Subsystem1 : Subsystem
  Transformation abc --> dq : Subsystem
  Vdc_ref (V) : Constant  Value=Vdc_nom
  Uctrl_grid_conv : Outport
  Vdqs : Outport  Port=2
  wires:
  Transformation abc --> dq/1(Vdq) -> Current regulator/1(Vdqs), Vdqs/1
  Theta/1 -> Transformation abc --> dq/1(Theta), Subsystem1/1(Theta)
  Vdc/1 -> Subsystem1/3(Vdc), DC bus voltage Regulator/2(Vdc)
  DC bus voltage Regulator/1(Id_ref) -> Mux/1
  Transformation abc --> dq/2(Idq) -> Current regulator/2(Idq)
  Mux/1 -> Idq references/1(Id*Iq*)
  Rate Limiter/1 -> Mux/2
  Iq_ref/1 -> Rate Limiter/1
  Vabc_B1/1 -> Transformation abc --> dq/2(Vabc)
  Iabc_grid_conv/1 -> Transformation abc --> dq/3(Iabc)
  Subsystem1/1(Uctrl_grid_conv) -> Uctrl_grid_conv/1
  Vdc_ref (V)/1 -> DC bus voltage Regulator/1(Vdc_ref)
  Current regulator/1(Vdq*) -> Subsystem1/2(Vdq*)
  Idq references/1(Idq_ref) -> Current regulator/4(Idq_ref)
  Freq/1 -> Current regulator/3(Freq)

== system SSN_39busRT_Ctrl_4WT_19B/SM_master/4 WT/SS_windfarm3to4/Wind Farm (DFIG Type)/Wind Turbine Doubly-Fed Induction Generator (Average Model)1/Control System_average/Control/Rotor-side converter Control system ==
  note: Rotor-side converter control system
  wr : Inport
  Vdc : Inport  Port=2
  Theta : Inport  Port=3
  Iabc_stator : Inport  Port=4
  Iabc_rotor : Inport  Port=5
  Iabc_grid_conv : Inport  Port=6
  Q_ref : Inport  Port=7
  Q_B1 : Inport  Port=8
  angle_rotor : Inport  Port=9
  Freq : Inport  Port=10
  Vdqs : Inport  Port=11
  Current Regulator : Subsystem
  Mux3 : Mux  Inputs=2
  Priority Iqr : Subsystem
  Q Regulator : Subsystem
  Torque control : Subsystem
  "Transformation abc --> dq " : Subsystem
  dq --> abc : Subsystem
  Uctrl_rotor_conv : Outport
  wires:
  Current Regulator/1(Vdq*) -> dq --> abc/1(Vdq*)
  Vdc/1 -> dq --> abc/2(Vdc)
  Theta/1 -> "Transformation abc --> dq "/1(Theta)
  dq --> abc/1(Uctrl_rotor_conv) -> Uctrl_rotor_conv/1
  Iabc_rotor/1 -> "Transformation abc --> dq "/2(Iabc_r)
  Iabc_stator/1 -> "Transformation abc --> dq "/3(Iabc_s)
  Iabc_grid_conv/1 -> "Transformation abc --> dq "/4(Iabc_grid_conv)
  "Transformation abc --> dq "/1(Idq_r) -> Current Regulator/2(Idq_r), Torque control/2(Idqr)
  "Transformation abc --> dq "/2(Idq_s) -> Torque control/3(Idqs), Current Regulator/3(Idq_s)
  angle_rotor/1 -> "Transformation abc --> dq "/5(angle_rotor)
  Mux3/1 -> Priority Iqr/1(Idqr*)
  "Transformation abc --> dq "/4(r_angle_transformation) -> dq --> abc/3(Angle)
  Freq/1 -> Torque control/5(Freq), Current Regulator/5(Freq)
  wr/1 -> Torque control/1(wr), Current Regulator/4(wr)
  "Transformation abc --> dq "/3(Idq_gc) -> Torque control/4(Idq_grid_conv)
  Vdqs/1 -> Torque control/6(Vdqs)
  Q_ref/1 -> Q Regulator/1(Q_ref)
  Q_B1/1 -> Q Regulator/2(Q_B1)
  Torque control/1(Idr*) -> Mux3/1
  Q Regulator/1(Iqr*) -> Mux3/2
  Priority Iqr/1(Idqr_ref) -> Current Regulator/1(Idqr_ref)

== system SSN_39busRT_Ctrl_4WT_19B/SM_master/4 WT/SS_windfarm3to4/Wind Farm (DFIG Type)2/Wind Turbine Doubly-Fed Induction Generator (Average Model)1/Average_VSC/Converter_model/Predictor ==
  In : Inport
  Add2 : Sum  Inputs=+-
  Gain1 : Gain  Gain=2
  Unit Delay : UnitDelay  SampleTime=Ts  HasFrameUpgradeWarning=on
  Out : Outport
  wires:
  Add2/1 -> Out/1
  Unit Delay/1 -> Add2/2
  Gain1/1 -> Add2/1
  In/1 -> Gain1/1, Unit Delay/1

== system SSN_39busRT_Ctrl_4WT_19B/SM_master/4 WT/SS_windfarm3to4/Wind Farm (DFIG Type)2/Wind Turbine Doubly-Fed Induction Generator (Average Model)1/Average_VSC1/Converter_model/Predictor ==
  In : Inport
  Add2 : Sum  Inputs=+-
  Gain1 : Gain  Gain=2
  Unit Delay : UnitDelay  SampleTime=Ts  HasFrameUpgradeWarning=on
  Out : Outport
  wires:
  Add2/1 -> Out/1
  Unit Delay/1 -> Add2/2
  Gain1/1 -> Add2/1
  In/1 -> Gain1/1, Unit Delay/1

== system SSN_39busRT_Ctrl_4WT_19B/SM_master/4 WT/SS_windfarm3to4/Wind Farm (DFIG Type)2/Wind Turbine Doubly-Fed Induction Generator (Average Model)1/Control System_average/Control/Grid-side converter Control system ==
  note: Grid-side converter control system
  Vabc_B1 : Inport
  Iabc_grid_conv : Inport  Port=2
  Theta : Inport  Port=3
  Vdc : Inport  Port=4
  Iq_ref : Inport  Port=5
  Freq : Inport  Port=6
  Current regulator : Subsystem
  DC bus voltage Regulator : Subsystem
  Idq references : Subsystem
  Mux : Mux  Inputs=2
  Rate Limiter : RateLimiter  RisingSlewLimit=current_slew_rate  FallingSlewLimit=-current_slew_rate
  Subsystem1 : Subsystem
  Transformation abc --> dq : Subsystem
  Vdc_ref (V) : Constant  Value=Vdc_nom
  Uctrl_grid_conv : Outport
  Vdqs : Outport  Port=2
  wires:
  Freq/1 -> Current regulator/3(Freq)
  Idq references/1(Idq_ref) -> Current regulator/4(Idq_ref)
  Current regulator/1(Vdq*) -> Subsystem1/2(Vdq*)
  Vdc_ref (V)/1 -> DC bus voltage Regulator/1(Vdc_ref)
  Subsystem1/1(Uctrl_grid_conv) -> Uctrl_grid_conv/1
  Iabc_grid_conv/1 -> Transformation abc --> dq/3(Iabc)
  Vabc_B1/1 -> Transformation abc --> dq/2(Vabc)
  Iq_ref/1 -> Rate Limiter/1
  Rate Limiter/1 -> Mux/2
  Mux/1 -> Idq references/1(Id*Iq*)
  Transformation abc --> dq/2(Idq) -> Current regulator/2(Idq)
  DC bus voltage Regulator/1(Id_ref) -> Mux/1
  Vdc/1 -> DC bus voltage Regulator/2(Vdc), Subsystem1/3(Vdc)
  Theta/1 -> Subsystem1/1(Theta), Transformation abc --> dq/1(Theta)
  Transformation abc --> dq/1(Vdq) -> Vdqs/1, Current regulator/1(Vdqs)

== system SSN_39busRT_Ctrl_4WT_19B/SM_master/4 WT/SS_windfarm3to4/Wind Farm (DFIG Type)2/Wind Turbine Doubly-Fed Induction Generator (Average Model)1/Control System_average/Control/Rotor-side converter Control system ==
  note: Rotor-side converter control system
  wr : Inport
  Vdc : Inport  Port=2
  Theta : Inport  Port=3
  Iabc_stator : Inport  Port=4
  Iabc_rotor : Inport  Port=5
  Iabc_grid_conv : Inport  Port=6
  Q_ref : Inport  Port=7
  Q_B1 : Inport  Port=8
  angle_rotor : Inport  Port=9
  Freq : Inport  Port=10
  Vdqs : Inport  Port=11
  Current Regulator : Subsystem
  Mux3 : Mux  Inputs=2
  Priority Iqr : Subsystem
  Q Regulator : Subsystem
  Torque control : Subsystem
  "Transformation abc --> dq " : Subsystem
  dq --> abc : Subsystem
  Uctrl_rotor_conv : Outport
  wires:
  Priority Iqr/1(Idqr_ref) -> Current Regulator/1(Idqr_ref)
  Q Regulator/1(Iqr*) -> Mux3/2
  Torque control/1(Idr*) -> Mux3/1
  Q_B1/1 -> Q Regulator/2(Q_B1)
  Q_ref/1 -> Q Regulator/1(Q_ref)
  Vdqs/1 -> Torque control/6(Vdqs)
  "Transformation abc --> dq "/3(Idq_gc) -> Torque control/4(Idq_grid_conv)
  wr/1 -> Current Regulator/4(wr), Torque control/1(wr)
  Freq/1 -> Current Regulator/5(Freq), Torque control/5(Freq)
  "Transformation abc --> dq "/4(r_angle_transformation) -> dq --> abc/3(Angle)
  Mux3/1 -> Priority Iqr/1(Idqr*)
  angle_rotor/1 -> "Transformation abc --> dq "/5(angle_rotor)
  "Transformation abc --> dq "/2(Idq_s) -> Current Regulator/3(Idq_s), Torque control/3(Idqs)
  "Transformation abc --> dq "/1(Idq_r) -> Torque control/2(Idqr), Current Regulator/2(Idq_r)
  Iabc_grid_conv/1 -> "Transformation abc --> dq "/4(Iabc_grid_conv)
  Iabc_stator/1 -> "Transformation abc --> dq "/3(Iabc_s)
  Iabc_rotor/1 -> "Transformation abc --> dq "/2(Iabc_r)
  dq --> abc/1(Uctrl_rotor_conv) -> Uctrl_rotor_conv/1
  Theta/1 -> "Transformation abc --> dq "/1(Theta)
  Vdc/1 -> dq --> abc/2(Vdc)
  Current Regulator/1(Vdq*) -> dq --> abc/1(Vdq*)

== system SSN_39busRT_Ctrl_4WT_19B/SM_master/4 WT/SS_windfarm1to2/Wind Farm (DFIG Type)/Wind Turbine Doubly-Fed Induction Generator (Average Model)1/Control System_average/Control/Grid-side converter Control system/Current regulator ==
  Vdqs : Inport
  Idq : Inport  Port=2
  Freq : Inport  Port=3
  Idq_ref : Inport  Port=4
  Constant1 : Constant  Value=L_RL
  Constant2 : Constant  Value=L_RL
  Constant3 : Constant  Value=R_RL
  Constant4 : Constant  Value=R_RL
  Demux{,1..3} (4 alike) : Demux  Outputs=2
      settings: DisplayOption=none
  Discrete PI Controller : powerlib_extras/Discrete  Control Blocks/Discrete PI Controller  Kp=Kpi_grid_side_cur_reg(1)  Ki=Kpi_grid_side_cur_reg(2)  Par_Limits=[1.1 -1.1]  Init=0  Ts=Ts_Control
  Divide3 : Product  Inputs=*/
  Fnom : Constant  Value=Fnom
  Mux : Mux  Inputs=2
  Mux1 : Mux  Inputs=2
  Product : Product  Inputs=3  InputSameDT=on  SaturateOnIntegerOverflow=on  OutDataTypeStr=Inherit: Same as first input
  Product1 : Product  Inputs=3  InputSameDT=on  SaturateOnIntegerOverflow=on  OutDataTypeStr=Inherit: Same as first input
  Product2 : Product  InputSameDT=on  SaturateOnIntegerOverflow=on  OutDataTypeStr=Inherit: Same as first input
  Product3 : Product  InputSameDT=on  SaturateOnIntegerOverflow=on  OutDataTypeStr=Inherit: Same as first input
  Sum1 : Sum  Inputs=|+-  InputSameDT=on  SaturateOnIntegerOverflow=on  OutDataTypeStr=Inherit: Same as first input
  Sum2 : Sum  Inputs=-+|  InputSameDT=on  SaturateOnIntegerOverflow=on  OutDataTypeStr=Inherit: Same as first input
  Sum3 : Sum  Inputs=||++-  InputSameDT=on  SaturateOnIntegerOverflow=on  OutDataTypeStr=Inherit: Same as first input
  Sum4 : Sum  Inputs=|+-  InputSameDT=on  SaturateOnIntegerOverflow=on  OutDataTypeStr=Inherit: Same as first input
  Sum5 : Sum  Inputs=|--+  InputSameDT=on  SaturateOnIntegerOverflow=on  OutDataTypeStr=Inherit: Same as first input
  Sum6 : Sum  Inputs=|-+  InputSameDT=on  SaturateOnIntegerOverflow=on  OutDataTypeStr=Inherit: Same as first input
  Vdq* : Outport
  wires:
  Constant2/1 -> Product1/2
  Demux3/1 -> Sum1/2  "vd'"
  Discrete PI Controller/1 -> Demux3/1
  Mux1/1 -> Discrete PI Controller/1
  Demux2/1 -> Sum3/1  "Vd"
  Constant1/1 -> Product/1
  Vdqs/1 -> Demux2/1
  Demux1/2 -> Sum2/2, [iqr]  "Iq_ref"
  Idq_ref/1 -> Demux1/1
  Demux1/1 -> Sum4/1, [idr]  "Id_ref"
  Demux/2 -> Sum2/1  "Iq"
  Demux/1 -> Sum4/2  "Id"
  Idq/1 -> Demux/1
  Sum6/1 -> Mux/2
  Sum1/1 -> Mux/1
  Mux/1 -> Vdq*/1
  Demux3/2 -> Sum6/1  "vq'"
  Product/1 -> Sum3/2
  Constant3/1 -> Product2/1
  Constant4/1 -> Product3/2
  Product1/1 -> Sum5/2
  Demux2/2 -> Sum5/3  "Vq"
  Product2/1 -> Sum3/3
  Product3/1 -> Sum5/1
  Sum5/1 -> Sum6/2
  Sum3/1 -> Sum1/1
  Sum4/1 -> Mux1/1
  Sum2/1 -> Mux1/2
  Freq/1 -> Divide3/1
  Fnom/1 -> Divide3/2
  Divide3/1 -> [w_pu]
  [w_pu] -> Product1/3
  [w_pu] -> Product/2
  [iqr] -> Product/3
  [idr] -> Product2/2
  [iqr] -> Product3/1
  [idr] -> Product1/1

== system SSN_39busRT_Ctrl_4WT_19B/SM_master/4 WT/SS_windfarm1to2/Wind Farm (DFIG Type)/Wind Turbine Doubly-Fed Induction Generator (Average Model)1/Control System_average/Control/Grid-side converter Control system/DC bus voltage Regulator ==
  Vdc_ref : Inport
  Vdc : Inport  Port=2
  Discrete PI Controller : powerlib_extras/Discrete  Control Blocks/Discrete PI Controller  Kp=Kpi_dc_reg(1)  Ki=Kpi_dc_reg(2)  Par_Limits=[1 -1]*Imax_grid_conv  Init=0  Ts=Ts_Control
  Rate Limiter : RateLimiter  RisingSlewLimit=current_slew_rate  FallingSlewLimit=-current_slew_rate
  Sum7 : Sum  Inputs=|+-  InputSameDT=on  SaturateOnIntegerOverflow=on  OutDataTypeStr=Inherit: Same as first input
  Id_ref : Outport
  wires:
  Sum7/1 -> Discrete PI Controller/1
  Vdc_ref/1 -> Sum7/1
  Discrete PI Controller/1 -> Rate Limiter/1
  Vdc/1 -> Sum7/2
  Rate Limiter/1 -> Id_ref/1

== system SSN_39busRT_Ctrl_4WT_19B/SM_master/4 WT/SS_windfarm1to2/Wind Farm (DFIG Type)/Wind Turbine Doubly-Fed Induction Generator (Average Model)1/Control System_average/Control/Grid-side converter Control system/Idq references ==
  Id*Iq* : Inport
  Cartesian to Polar : simulink_extras/Transformations/Cartesian to Polar
  Demux : Demux  Outputs=2
      settings: DisplayOption=none
  Igrid_conv_max^2 : Constant  Value=Imax_grid_conv^2
  Math Function : Math  Operator=square  SignedPower=on  SaturateOnIntegerOverflow=on
  Math Function1 : Math  Operator=sqrt  SignedPower=on  SaturateOnIntegerOverflow=on
  Mux : Mux  Inputs=2
  Mux1 : Mux  Inputs=2
  Product : Product  InputSameDT=on  SaturateOnIntegerOverflow=on  OutDataTypeStr=Inherit: Same as first input
  Rate Limiter : RateLimiter  RisingSlewLimit=current_slew_rate  FallingSlewLimit=-current_slew_rate
  Sign : Signum  ZeroCross=off
  Sum : Sum  Inputs=|+-  InputSameDT=on  SaturateOnIntegerOverflow=on  OutDataTypeStr=Inherit: Same as first input
  Switch : Switch  Threshold=Imax_grid_conv  SaturateOnIntegerOverflow=on  InputSameDT=on
  Terminator : Terminator
  Idq_ref : Outport
  wires:
  Id*Iq*/1 -> Demux/1
  Sign/1 -> Product/1
  Math Function1/1 -> Product/2  "Iq"
  Switch/1 -> Rate Limiter/1
  Mux1/1 -> Switch/1
  Sum/1 -> Math Function1/1
  Math Function/1 -> Sum/2
  Igrid_conv_max^2/1 -> Sum/1
  Mux/1 -> Switch/3
  Cartesian to Polar/1 -> Switch/2
  Cartesian to Polar/2 -> Terminator/1
  Demux/1 -> Mux/1, Cartesian to Polar/1, Math Function/1, Mux1/1
  Demux/2 -> Sign/1, Mux/2, Cartesian to Polar/2
  Rate Limiter/1 -> Idq_ref/1
  Product/1 -> Mux1/2

== system SSN_39busRT_Ctrl_4WT_19B/SM_master/4 WT/SS_windfarm1to2/Wind Farm (DFIG Type)/Wind Turbine Doubly-Fed Induction Generator (Average Model)1/Control System_average/Control/Grid-side converter Control system/Subsystem1 ==
  note: Required value for modulation index "m" to obtain 1 pu generated voltage by the converter:
  note: m = Vnom * 2*sqrt(2/3) / Vdc
  note: Where Vnom = RMS ph-ph nominal voltage
  Theta : Inport
  Vdq* : Inport  Port=2
  Vdc : Inport  Port=3
  0-1 : Saturate  UpperLimit=1  LowerLimit=0
  Avoid division by zero : Saturate  UpperLimit=1e6  LowerLimit=1e-6
  Cartesian to Polar1 : simulink_extras/Transformations/Cartesian to Polar
  Demux1 : Demux  Outputs=2
      settings: DisplayOption=none
  K : Constant  Value=Vnom*2*sqrt(2/3)
  Mux : Mux  Inputs=3
  Mux1 : Mux  Inputs=2
  Polar to Cartesian : simulink_extras/Transformations/Polar to Cartesian
      settings: SourceProductBaseCode=SL
  Product1 : Product  Inputs=**/  InputSameDT=on  SaturateOnIntegerOverflow=on  OutDataTypeStr=Inherit: Same as first input
  Trigonometric Function2 : Trigonometry
  Trigonometric Function3 : Trigonometry  Operator=cos
  V0 : Constant  Value=0
  dq0_to_abc Transformation : powerlib_extras/Measurements/dq0_to_abc Transformation
      settings: SourceProductBaseCode=PS
  Uctrl_grid_conv : Outport
  wires:
  Mux1/1 -> dq0_to_abc Transformation/2
  Trigonometric Function2/1 -> Mux1/1
  Trigonometric Function3/1 -> Mux1/2
  V0/1 -> Mux/3
  dq0_to_abc Transformation/1 -> Uctrl_grid_conv/1
  Polar to Cartesian/1 -> Mux/1
  Polar to Cartesian/2 -> Mux/2
  Mux/1 -> dq0_to_abc Transformation/1  "Vdq0"
  0-1/1 -> Polar to Cartesian/1
  Product1/1 -> 0-1/1  "m"
  Vdc/1 -> Avoid division by zero/1
  K/1 -> Product1/2
  Avoid division by zero/1 -> Product1/3
  Vdq*/1 -> Demux1/1
  Theta/1 -> Trigonometric Function2/1, Trigonometric Function3/1
  Demux1/1 -> Cartesian to Polar1/1
  Demux1/2 -> Cartesian to Polar1/2
  Cartesian to Polar1/1 -> Product1/1
  Cartesian to Polar1/2 -> Polar to Cartesian/2

== system SSN_39busRT_Ctrl_4WT_19B/SM_master/4 WT/SS_windfarm1to2/Wind Farm (DFIG Type)/Wind Turbine Doubly-Fed Induction Generator (Average Model)1/Control System_average/Control/Grid-side converter Control system/Transformation abc --> dq ==
  Theta : Inport
  Vabc : Inport  Port=2
  Iabc : Inport  Port=3
  Demux1 : Demux  Outputs=[2 1]
      settings: DisplayOption=none
  Demux3 : Demux  Outputs=[2 1]
      settings: DisplayOption=none
  Mux1 : Mux  Inputs=2
  Terminator1 : Terminator
  Terminator3 : Terminator
  Trigonometric Function2 : Trigonometry
  Trigonometric Function3 : Trigonometry  Operator=cos
  abc_to_dq0 : powerlib_extras/Measurements/abc_to_dq0 Transformation
      settings: SourceProductBaseCode=PS
  "abc_to_dq0  " : powerlib_extras/Measurements/abc_to_dq0 Transformation
      settings: SourceProductBaseCode=PS
  Vdq : Outport
  Idq : Outport  Port=2
  wires:
  Theta/1 -> Trigonometric Function3/1, Trigonometric Function2/1
  abc_to_dq0/1 -> Demux3/1
  Vabc/1 -> abc_to_dq0/1
  "abc_to_dq0  "/1 -> Demux1/1
  Trigonometric Function2/1 -> Mux1/1
  Trigonometric Function3/1 -> Mux1/2
  Mux1/1 -> "abc_to_dq0  "/2, abc_to_dq0/2
  Demux3/2 -> Terminator3/1
  Demux3/1 -> Vdq/1
  Demux1/2 -> Terminator1/1
  Demux1/1 -> Idq/1
  Iabc/1 -> "abc_to_dq0  "/1
